simulink model "RetinaSathiScreeningWorkflow"  (R2026a)
settings: Solver=VariableStepDiscrete  StopTime=480
undefined symbols (not defined in the file or in its folder): m, n
settings Model: Creator=mddanish  LastModifiedBy=mddanish

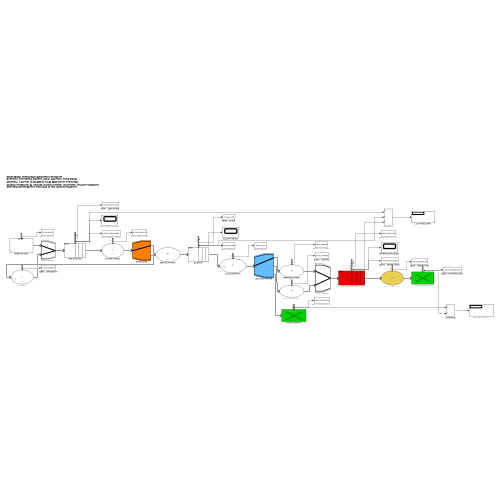
[thumbnail: Simulink's stored preview of the top-level diagram]
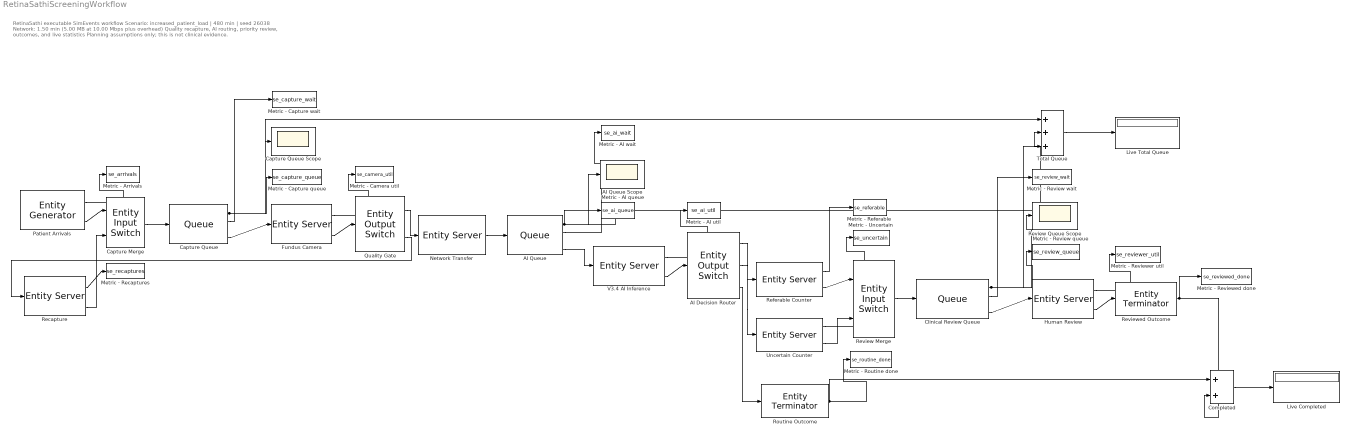
== system RetinaSathiScreeningWorkflow ==
  note: RetinaSathi executable SimEvents workflow
      | Scenario: increased_patient_load | 480 min | seed 26038
      | Network: 1.50 min (5.00 MB at 10.00 Mbps plus overhead)
      | Quality recapture, AI routing, priority review, outcomes, and live statistics
      | Planning assumptions only; this is not clinical evidence.
  AI Decision Router : EntityOutputSwitch  InputPortMessageModes=m  OutputPortMessageModes=m,m,m  NumberOutputPorts=3  SwitchingCriterion=From attribute  SwitchAttributeName=route
      settings: OutputPortMap=o0,o1,o2
  AI Queue : Queue  InputPortMessageModes=m  OutputPortMessageModes=n,n,n,m  Capacity=inf  NumberEntitiesInBlock=on  AverageWait=on  AverageQueueLength=on
      settings: OutputPortMap=o1,o2,o3,o5
  AI Queue Scope : Scope
  Capture Merge : EntityInputSwitch  InputPortMessageModes=m,m  OutputPortMessageModes=m
  Capture Queue : Queue  InputPortMessageModes=m  OutputPortMessageModes=n,n,n,m  Capacity=inf  NumberEntitiesInBlock=on  AverageWait=on  AverageQueueLength=on
      settings: OutputPortMap=o1,o2,o3,o5
  Capture Queue Scope : Scope
  Clinical Review Queue : Queue  InputPortMessageModes=m  OutputPortMessageModes=n,n,n,m  Capacity=inf  NumberEntitiesInBlock=on  AverageWait=on  AverageQueueLength=on
      settings: OutputPortMap=o1,o2,o3,o5
  Completed : Sum
  Fundus Camera : EntityServer  InputPortMessageModes=m  OutputPortMessageModes=n,m  Capacity=1  ServiceTimeValue=6  Utilization=on
      settings: OutputPortMap=o5,o9
  Human Review : EntityServer  InputPortMessageModes=m  OutputPortMessageModes=n,m  Capacity=1  ServiceTimeValue=8  Utilization=on
      settings: OutputPortMap=o5,o9
  Live Completed : Display
  Live Total Queue : Display
  Metric - AI queue : ToWorkspace  VariableName=se_ai_queue  SaveFormat=Timeseries  SampleTime=-1
  Metric - AI util : ToWorkspace  VariableName=se_ai_util  SaveFormat=Timeseries  SampleTime=-1
  Metric - AI wait : ToWorkspace  VariableName=se_ai_wait  SaveFormat=Timeseries  SampleTime=-1
  Metric - Arrivals : ToWorkspace  VariableName=se_arrivals  SaveFormat=Timeseries  SampleTime=-1
  Metric - Camera util : ToWorkspace  VariableName=se_camera_util  SaveFormat=Timeseries  SampleTime=-1
  Metric - Capture queue : ToWorkspace  VariableName=se_capture_queue  SaveFormat=Timeseries  SampleTime=-1
  Metric - Capture wait : ToWorkspace  VariableName=se_capture_wait  SaveFormat=Timeseries  SampleTime=-1
  Metric - Recaptures : ToWorkspace  VariableName=se_recaptures  SaveFormat=Timeseries  SampleTime=-1
  Metric - Referable : ToWorkspace  VariableName=se_referable  SaveFormat=Timeseries  SampleTime=-1
  Metric - Review queue : ToWorkspace  VariableName=se_review_queue  SaveFormat=Timeseries  SampleTime=-1
  Metric - Review wait : ToWorkspace  VariableName=se_review_wait  SaveFormat=Timeseries  SampleTime=-1
  Metric - Reviewed done : ToWorkspace  VariableName=se_reviewed_done  SaveFormat=Timeseries  SampleTime=-1
  Metric - Reviewer util : ToWorkspace  VariableName=se_reviewer_util  SaveFormat=Timeseries  SampleTime=-1
  Metric - Routine done : ToWorkspace  VariableName=se_routine_done  SaveFormat=Timeseries  SampleTime=-1
  Metric - Uncertain : ToWorkspace  VariableName=se_uncertain  SaveFormat=Timeseries  SampleTime=-1
  Network Transfer : EntityServer  InputPortMessageModes=m  OutputPortMessageModes=m  Capacity=Inf  ServiceTimeValue=1.5
  Patient Arrivals : EntityGenerator  OutputPortMessageModes=n,m  TimeSource=MATLAB action  IntergenerationTimeAction=persistent state; if isempty(state), state = 26038; end; state = mod(16807*state,2147483647); u = max(double(state)/2147483647,1e-12); dt = -log(u)/0.22;  GenerateEntityAtSimulationStart=off  GenerateAction=u = mod(double(entitySys.id)*7919 + 26038,10000)/10000; if u < 0.12, entity.route = 2; else, entity.route = 1; end;  AttributeName=route  NumberEntitiesDeparted=on  EntityType=Structured  EntityTypeName=Entity
      settings: OutputPortMap=o0,o3
  Quality Gate : EntityOutputSwitch  InputPortMessageModes=m  OutputPortMessageModes=m,m  SwitchingCriterion=From attribute  SwitchAttributeName=route
  Recapture : EntityServer  InputPortMessageModes=m  OutputPortMessageModes=n,m  Capacity=1  ServiceTimeValue=6  ServiceCompleteAction=entity.route = 1;  NumberEntitiesDeparted=on
      settings: OutputPortMap=o0,o9
  Referable Counter : EntityServer  InputPortMessageModes=m  OutputPortMessageModes=n,m  Capacity=Inf  ServiceTimeValue=0  NumberEntitiesDeparted=on
      settings: OutputPortMap=o0,o9
  Review Merge : EntityInputSwitch  InputPortMessageModes=m,m  OutputPortMessageModes=m
  Review Queue Scope : Scope
  Reviewed Outcome : EntityTerminator  InputPortMessageModes=m  NumberEntitiesArrived=on
      settings: OutputPortMap=o0
  Routine Outcome : EntityTerminator  InputPortMessageModes=m  NumberEntitiesArrived=on
      settings: OutputPortMap=o0
  Total Queue : Sum  Inputs=+++
  Uncertain Counter : EntityServer  InputPortMessageModes=m  OutputPortMessageModes=n,m  Capacity=Inf  ServiceTimeValue=0  NumberEntitiesDeparted=on
      settings: OutputPortMap=o0,o9
  V3.4 AI Inference : EntityServer  InputPortMessageModes=m  OutputPortMessageModes=n,m  Capacity=1  ServiceTimeValue=1.2  ServiceCompleteAction=u1 = mod(double(entitySys.id)*3571 + 26055,10000)/10000; u2 = mod(double(entitySys.id)*6271 + 26069,10000)/10000; u3 = mod(double(entitySys.id)*4513 + 26085,10000)/10000; if u1 < 0.28, entity.route = 1; if u3 < 0.25, entitySys.priority = 1; else, entitySys.priority = 2; end; elseif u2 < 0.1, entity.route = 2; entitySys.priority = 3; else, entity.route = 3; entitySys.priority = 4; end;  Utilization=on
      settings: OutputPortMap=o5,o9
  wires:
  Completed/1 -> Live Completed/1
  Total Queue/1 -> Live Total Queue/1
  Clinical Review Queue/4 -> Human Review/1
  Clinical Review Queue/2 -> Metric - Review wait/1
  Review Merge/1 -> Clinical Review Queue/1
  Routine Outcome/1 -> Metric - Routine done/1, Completed/1
  Uncertain Counter/2 -> Review Merge/2
  Uncertain Counter/1 -> Metric - Uncertain/1
  AI Decision Router/3 -> Routine Outcome/1
  AI Decision Router/2 -> Uncertain Counter/1
  AI Queue/4 -> V3.4 AI Inference/1
  AI Queue/2 -> Metric - AI wait/1
  Network Transfer/1 -> AI Queue/1
  V3.4 AI Inference/1 -> Metric - AI util/1
  Clinical Review Queue/1 -> Review Queue Scope/1, Metric - Review queue/1, Total Queue/3
  AI Queue/1 -> AI Queue Scope/1, Metric - AI queue/1, Total Queue/2
  Reviewed Outcome/1 -> Completed/2, Metric - Reviewed done/1
  Quality Gate/2 -> Recapture/1
  Quality Gate/1 -> Network Transfer/1
  Referable Counter/1 -> Metric - Referable/1
  Capture Queue/4 -> Fundus Camera/1
  Fundus Camera/2 -> Quality Gate/1
  V3.4 AI Inference/2 -> AI Decision Router/1
  Capture Merge/1 -> Capture Queue/1
  Human Review/2 -> Reviewed Outcome/1
  Fundus Camera/1 -> Metric - Camera util/1
  Human Review/1 -> Metric - Reviewer util/1
  Capture Queue/1 -> Capture Queue Scope/1, Metric - Capture queue/1, Total Queue/1
  AI Decision Router/1 -> Referable Counter/1
  Capture Queue/2 -> Metric - Capture wait/1
  Referable Counter/2 -> Review Merge/1
  Patient Arrivals/1 -> Metric - Arrivals/1
  Recapture/2 -> Capture Merge/2
  Recapture/1 -> Metric - Recaptures/1
  Patient Arrivals/2 -> Capture Merge/1
